simulink model "Team2_Demo1Simulink391"  (R2023b)
settings: Solver=VariableStepAuto  StartTime=0.0  StopTime=60  RelTol=1e-3
undefined symbols (not defined in the file): QAM
libraries: commchan3 x2, simulink x2, commcnvcod2 x2, dspvision x2, commfilt2 x2, commdigbbndam3 x2, dspquant2 x2, dspsnks4 x1, commsink2 x1
settings Model: Creator=weiyang  LastModifiedBy=bryan

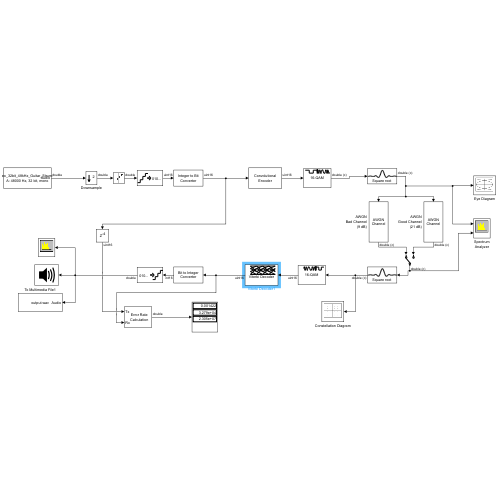
[thumbnail: Simulink's stored preview of the top-level diagram]
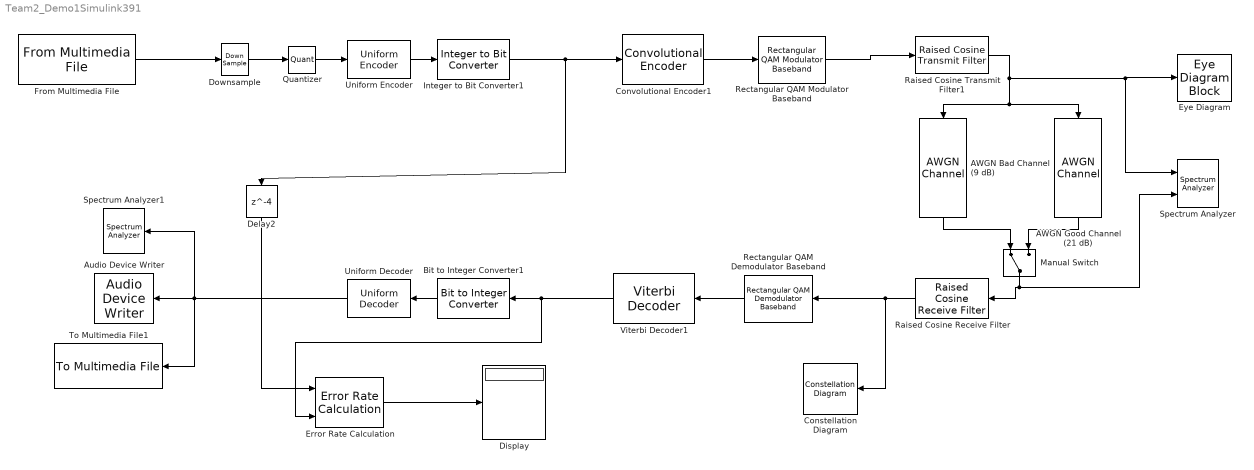
== system Team2_Demo1Simulink391 ==
  AWGN Bad Channel (9 dB) : commchan3/AWGN Channel  LegacyMode=off  NoiseMethod="Signal to noise ratio  (SNR)"  noiseMode="Signal to noise ratio  (SNR)"  EbNo=9  EsNo=10  SNR=9  BitsPerSymbol=1  SignalPower=1  SamplesPerSymbol=1  SymbolPeriod=1  VarianceSource=Parameter  Variance=1  RandomStream=Global stream  Seed=67  SimulateUsing=Code generation
  AWGN Good Channel (21 dB) : commchan3/AWGN Channel  LegacyMode=off  NoiseMethod="Signal to noise ratio  (SNR)"  noiseMode="Signal to noise ratio  (SNR)"  EbNo=10  EsNo=10  SNR=21  BitsPerSymbol=1  SignalPower=1  SamplesPerSymbol=1  SymbolPeriod=1  VarianceSource=Parameter  Variance=1  RandomStream=Global stream  Seed=67  SimulateUsing=Code generation
  Audio Device Writer : dspsnks4/Audio Device Writer  Driver=DirectSound  Device=Default  InheritSampleRate=on  SampleRate=44100  BitDepth=16-bit integer  BufferSize=4096  NumBuffers=10  DefaultOutputChannelMapping=on  OutputChannelMapping=1:2  OutputNumUnderrunSamples=off  DriverIdx=1  DeviceWarnFlag=''
  Bit to Integer Converter1 : simulink/Logic and Bit Operations/Bit to Integer Converter  nbits=16  bitOrder=MSB first  signedOutputValues=Signed  outDtype=uint16  outDtypeSigned=int16
  Constellation Diagram : ConstellationDiagram  WindowPosition=[505.000000,151.000000,736.000000,600.000000,]  Visible=on  ScopeFrameLocation=window  ReferenceConstellation=16-QAM
  Convolutional Encoder1 : commcnvcod2/Convolutional Encoder  trellis=poly2trellis(7, [171 133])  opMode=Continuous  DelayedResetAction=off  hasIniStPort=off  hasFinStPort=off  usePuncVector=off  punctureVector=[1; 1; 0; 1; 0; 1]  reset=Unused parameter value
  Delay2 : Delay  DelayLength=4
  Display : Display
  Downsample : DownSample  RateOptions=Allow multirate processing
  Error Rate Calculation : commsink2/Error Rate Calculation  N=34  st_delay=0  cp_mode=Entire frame  subframe=[]  PMode=Port  WsName=ErrorVec  RsMode2=off  stop=off  numErr=100  maxBits=1e6
      settings: LibrarySourceBlock=|
      | commhdlsink/Error Rate
      | Calculation
  Eye Diagram : EyeDiagramBlock  WindowPosition=[368.000000,182.000000,800.000000,500.000000,]  Visible=on  ScopeFrameLocation=window
  From Multimedia File : dspvision/From Multimedia File  inputFilename=C:\Users\bryan\Downloads\ELEC 391\Assignments\ELEC391_Sound_Files\Stereo_32bit_48kHz_Guitar_Strum.wav  readRange=[1 Inf]  loop=on  numPlays=inf  outputStreams=Audio only  videoDataType=single  audioDataType=double  inheritSampleTime=on  userDefinedSampleTime=1/30  noAudioOutput=off  isIntensityVideo=off  fourcc=RGB  colorVideoFormat=Separate color signals  outputEOF=off  dataOrg=Column-major  audioFrameSize=1024  computeAudioFrameSize=off  outSamplingMode=Sample based
      settings: LibrarySourceBlock=audiosources/From Multimedia File
  Integer to Bit Converter1 : simulink/Logic and Bit Operations/Integer to Bit Converter  nbits=16  signedInputValues=Unsigned  bitOrder=MSB first  outDtype=uint16
  Manual Switch : ManualSwitch
  Quantizer : Quantizer  QuantizationInterval=0.0625
  Raised Cosine Receive Filter : commfilt2/Raised Cosine Receive Filter  filtType=Square root  R=0.2  filtSpan=4  N=10  downFactor=10  downOffset=0  filterGain=1  RateOptions=Allow multirate processing  framing=Mute  checkCoeff=off  variableName=rcRxFilt  currentFiltSpan=10  D=5  inputOffset=0  sampMode=Mute  saveAsFlag=0  rateMode=Downsampling  checkGain=Normalized  launchFVT=on  roundingMode=Floor  overflowMode=off  coeffDataTypeStr=Inherit: Same word length as input  coeffMin=[]  coeffMax=[]  coeffLastDataTypeStr=Inherit: Same word length as input  accumDataTypeStr=Inherit: Same as product output  accumLastDataTypeStr=Inherit: Same as product output  outputDataTypeStr=Inherit: Same as accumulator  outputMin=[]  outputMax=[]  outputLastDataTypeStr=Inherit: Same as accumulator
      settings: LibrarySourceBlock=|
      | commhdlfilt/Raised Cosine
      | Receive Filter
  Raised Cosine Transmit Filter1 : commfilt2/Raised Cosine Transmit Filter  filtType=Square root  R=0.2  filtSpan=4  N=10  filterGain=1  RateOptions=Allow multirate processing  framing=Mute  checkCoeff=off  variableName=rcTxFilt1  checkGain=Normalized  sampMode=Mute  saveAsFlag=0  currentFiltSpan=10  D=(10)/2  launchFVT=on  roundingMode=Floor  overflowMode=off  coeffDataTypeStr=Inherit: Same word length as input  coeffMin=[]  coeffMax=[]  coeffLastDataTypeStr=Inherit: Same word length as input  outputDataTypeStr=Inherit: Same as accumulator  outputMin=[]  outputMax=[]  outputLastDataTypeStr=Inherit: Same as accumulator
  Rectangular QAM Demodulator Baseband : commdigbbndam3/Rectangular QAM Demodulator Baseband  M=16  OutType=Bit  DecType=Hard decision  VarSource=Dialog  Variance=1  Dec=Gray  Mapping=[0:15]  PowType=Min. distance between symbols  MinDist=2  AvgPow=1  PeakPow=1  Ph=0  outDtype1=uint16  outDtype2=Inherit via internal rule  derotateFactorWordLen=16  derotateFactorDataTypeStr=Inherit: Same word length as input  derotateFactorLastDataTypeStr=Inherit: Same word length as input  denormFactorWordLen=16  denormFactorDataTypeStr=Inherit: Same word length as input  denormFactorLastDataTypeStr=Inherit: Same word length as input  prodOutWordLen=32  prodOutOverflowMode=Wrap  prodOutRoundingMode=Floor  prodOutOvFlMode=off  prodOutOvFlModeLastStrValue=off  sumWordLen=32
      settings: LibrarySourceBlock=|
      | commhdldigbbndam/Rectangular QAM
      | Demodulator
      | Baseband
  Rectangular QAM Modulator Baseband : commdigbbndam3/Rectangular QAM Modulator Baseband  M=16  InType=Bit  Enc=Gray  Mapping=[0:15]  PowType=Min. distance between symbols  MinDist=2  AvgPow=1  PeakPow=1  Ph=0  outDtype=double  outWordLen=16  outUDDataType=sfix(16)  outFracLenMode=Best precision  outFracLen=15  outDataTypeStr=double  outLastDataTypeStr=double
      settings: LibrarySourceBlock=|
      | commhdldigbbndam/Rectangular QAM
      | Modulator
      | Baseband
  Spectrum Analyzer : SpectrumAnalyzer  NumInputPorts=2  WindowPosition=[1.000000,49.000000,1539.000000,844.000000,]  Visible=on  ScopeFrameLocation=window  FrequencySpan=Span and center frequency  Span=12000  StartFrequency=-420000  StopFrequency=420000  YLimits=[-47.71617066,32.07283337]  ColorLimits=[-20 80]  ShowLegend=on  DefaultConfigurationName=spbscopes.SpectrumAnalyzerBlockCfg  IsFrequencyInputMode=0  FrequencyVectorPort=0  FrequencyVectorFromPort=0  FrequencyInputRBWPort=0  FrequencyInputRBWFromPort=0
  Spectrum Analyzer1 : SpectrumAnalyzer  WindowPosition=[301.000000,253.000000,800.000000,500.000000,]  Visible=on  ScopeFrameLocation=window  YLimits=[-62.98536533,26.96332919]  SelectedToolstripTab=spectrumAnalyzerToolstrip.spectralMaskTab
  To Multimedia File1 : dspvision/To Multimedia File  outputFilename=C:\Users\bryan\Downloads\ELEC 391\Assignments\output.wav  streamSelection=Audio only  videoCompressor=None (uncompressed)  audioCompressor=None (uncompressed)  imagePorts=One multidimensional signal  fileType=WAV  audioDatatype=16-bit integer  fourcc=RGB  videoQuality=75  mj2000CompFactor=10
      settings: LibrarySourceBlock=dspsnks4/To Multimedia File
  Uniform Decoder : dspquant2/Uniform Decoder  peak=1  bits=16  overflowMode=Saturate  otype=Double
  Uniform Encoder : dspquant2/Uniform Encoder  peak=1  bits=16  otype=Unsigned integer
  Viterbi Decoder1 : commcnvcod2/Viterbi Decoder  trellis=poly2trellis(7, [171 133])  isPunctured=off  punctureVector=[1; 1; 0; 1; 0; 1]  erasures=off  dectype=Hard decision  nsdecb=4  runSigValErrCheck=off  tbdepth=34  opmode=Continuous  reset=off  delayedResetAction=off  smWordLength=16  outDataType=uint16
  wires:
  Error Rate Calculation/1 -> Display/1
  Raised Cosine Transmit Filter1/1 -> Eye Diagram/1, Spectrum Analyzer/1, AWGN Bad Channel (9 dB)/1, AWGN Good Channel (21 dB)/1
  Delay2/1 -> Error Rate Calculation/1
  Viterbi Decoder1/1 -> Error Rate Calculation/2, Bit to Integer Converter1/1
  Uniform Decoder/1 -> Spectrum Analyzer1/1, Audio Device Writer/1, To Multimedia File1/1
  Uniform Encoder/1 -> Integer to Bit Converter1/1
  From Multimedia File/1 -> Downsample/1
  Raised Cosine Receive Filter/1 -> Rectangular QAM Demodulator Baseband/1, Constellation Diagram/1
  Manual Switch/1 -> Raised Cosine Receive Filter/1, Spectrum Analyzer/2
  AWGN Bad Channel (9 dB)/1 -> Manual Switch/1
  AWGN Good Channel (21 dB)/1 -> Manual Switch/2
  Rectangular QAM Demodulator Baseband/1 -> Viterbi Decoder1/1
  Convolutional Encoder1/1 -> Rectangular QAM Modulator Baseband/1
  Downsample/1 -> Quantizer/1
  Quantizer/1 -> Uniform Encoder/1
  Integer to Bit Converter1/1 -> Convolutional Encoder1/1, Delay2/1
  Bit to Integer Converter1/1 -> Uniform Decoder/1
  Rectangular QAM Modulator Baseband/1 -> Raised Cosine Transmit Filter1/1
